simulink model "teste.sil2"  (R2013a)
settings: Solver=ode1  StartTime=0.0  StopTime=10.0  RelTol=1e-3
libraries: simulink_extras x1
settings Model: Creator=amarc  LastModifiedBy=amarc

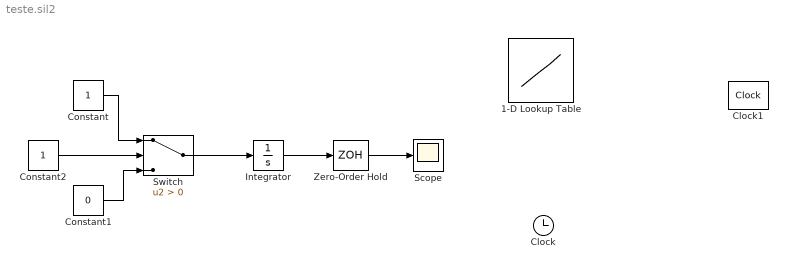
== system teste.sil2 ==
  1-D Lookup Table : Lookup_n-D  NumberOfTableDimensions=1  BreakpointsForDimension1=[-5:5]  Table=tanh([-5:5])  RndMeth=Simplest  InputSameDT=on
  Clock : Clock
  Clock1 : simulink_extras/Flip Flops/Clock  period=2
  Constant : Constant
  Constant1 : Constant  Value=0
  Constant2 : Constant
  Integrator : Integrator
  Scope : Scope
  Switch : Switch  Criteria=u2 > Threshold
  Zero-Order Hold : ZeroOrderHold
  wires:
  Integrator/1 -> Zero-Order Hold/1
  Zero-Order Hold/1 -> Scope/1
  Switch/1 -> Integrator/1
  Constant1/1 -> Switch/3
  Constant/1 -> Switch/1
  Constant2/1 -> Switch/2
